simulink model "FM_PLL_2022b"  (R2022b)
settings: Solver=ode45  StartTime=0.0  StopTime=0.0475*100  RelTol=1e-3  EnableMultiTasking=on
PreLoadFcn:
  | fm=15;
libraries: commsynccomp2 x2, dsparch4 x1
settings Model: Creator=morelos_zaragoza  LastModifiedBy=14083
settings SolverCC: AlgebraicLoopSolver=TrustRegion
settings DataIOCC: LimitDataPoints=on  SaveFormat=Array  SignalLoggingSaveFormat=ModelDataLogs  ReturnWorkspaceOutputs=off
settings OptimizationCC: ExpressionDepthLimit=2147483647  InitFltsAndDblsToZero=on  LifeSpan=inf
settings DebuggingCC: SaveWithParameterizedLinksMsg=none  UnderspecifiedInitializationDetection=Classic  MergeDetectMultiDrivingBlocksExec=none  SignalResolutionControl=TryResolveAllWithWarning  SolverPrmCheckMsg=warning  MultiTaskDSMMsg=warning  MultiTaskCondExecSysMsg=none  FcnCallInpInsideContextMsg=warning  UnconnectedInputMsg=warning  UnconnectedOutputMsg=warning  UnconnectedLineMsg=warning  StateNameClashWarn=warning  SFUnexpectedBacktrackingDiag=warning  SFNoUnconditionalDefaultTransitionDiag=warning  SFExecutionAtInitializationDiag=none  SFMachineParentedDataDiag=warning  ArithmeticOperatorsInVariantConditions=warning
settings HardwareCC: ProdBitPerPointer=32  ProdBitPerSizeT=32  ProdBitPerPtrDiffT=32  ProdLargestAtomicFloat=None  ProdIntDivRoundTo=Undefined  ProdEndianess=Unspecified  ProdWordSize=32  ProdHWDeviceType=32-bit Generic
settings ModelReferenceCC: EnableRefExpFcnMdlSchedulingChecks=on  PropagateSignalLabelsOutOfModel=off
settings SFSimCC: SimUseLocalCustomCode=off  CustomCodeUndefinedFunction=UseInterfaceOnly
settings RTWCC: RTWUseLocalCustomCode=off  DLArmComputeVersion=19.05
settings CodeAppCC: StateflowObjectComments=on
settings GRTTargetCC: TargetFcnLib=ansi_tfl_tmw.mat  TargetLangStandard=C89/C90 (ANSI)  CombineOutputUpdateFcns=off  GRTInterface=on
settings ConfigComp: CovMetricSettings=dw  CovSaveCumulativeToWorkspaceVar=on  CovSaveSingleToWorkspaceVar=on  CovExternalEMLEnable=off

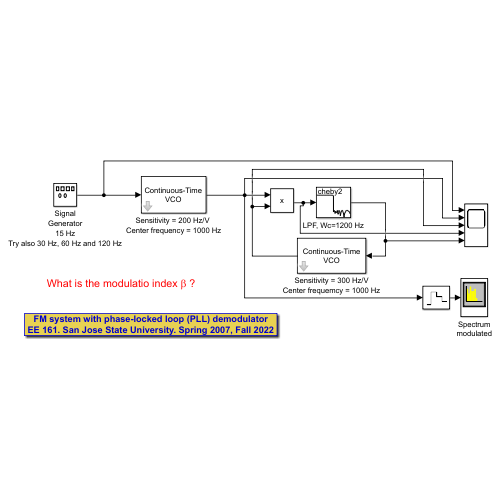
[thumbnail: Simulink's stored preview of the top-level diagram]
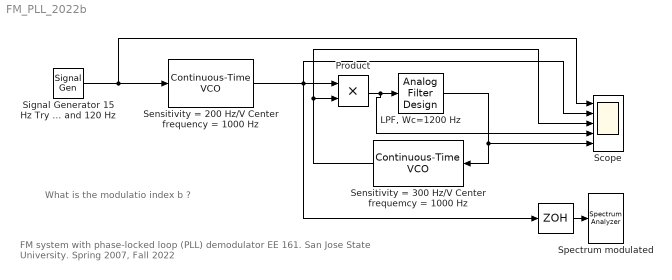
== system FM_PLL_2022b ==
  note: What is the modulatio index b ?
  note: FM system with phase-locked loop (PLL) demodulator
      | EE 161. San Jose State University. Spring 2007, Fall 2022
  "   " : ZeroOrderHold  SampleTime=1/4096
  "LPF, Wc=1200 Hz" : dsparch4/Analog Filter Design  method=Chebyshev II  filttype=Lowpass  N=20  Wlo=2*pi*1200  Whi=2*pi*110  Rp=2  Rs=40
  Product : Product  RndMeth=Zero
  Scope : Scope  NumInputPorts=5
  Sensitivity = 200 Hz/V Center frequency = 1000 Hz : commsynccomp2/Continuous-Time VCO  Ac=1  Fc=1000  Kc=200  Ph=0
  Sensitivity = 300 Hz/V Center frequemcy = 1000 Hz : commsynccomp2/Continuous-Time VCO  Ac=2  Fc=1000  Kc=300  Ph=0
  "Signal Generator 15 Hz Try also 30 Hz, 60 Hz and 120 Hz" : SignalGenerator  Frequency=fm
  Spectrum modulated : SpectrumAnalyzer
  wires:
  "Signal Generator 15 Hz Try also 30 Hz, 60 Hz and 120 Hz"/1 -> Sensitivity = 200 Hz/V Center frequency = 1000 Hz/1, Scope/1
  Sensitivity = 200 Hz/V Center frequency = 1000 Hz/1 -> Product/1, "   "/1, Scope/2
  Sensitivity = 300 Hz/V Center frequemcy = 1000 Hz/1 -> Scope/3, Product/2
  Product/1 -> Scope/4, "LPF, Wc=1200 Hz"/1
  "LPF, Wc=1200 Hz"/1 -> Scope/5, Sensitivity = 300 Hz/V Center frequemcy = 1000 Hz/1
  "   "/1 -> Spectrum modulated/1
